simulink model "DualMIPS_sim2_amartya"  (R2025a)
settings: Solver=FixedStepDiscrete  StartTime=0  StopTime=200  FixedStep=1  RelTol=1e-3
libraries: simulink_extras x2, hdlsllib x2
settings Model: Creator=amartyaraoponugoti  LastModifiedBy=prath

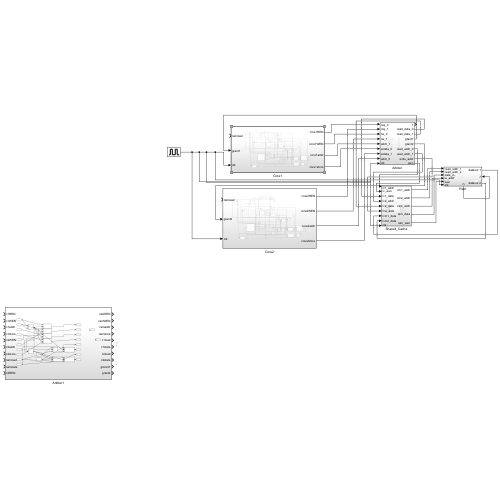
[thumbnail: Simulink's stored preview of the top-level diagram]
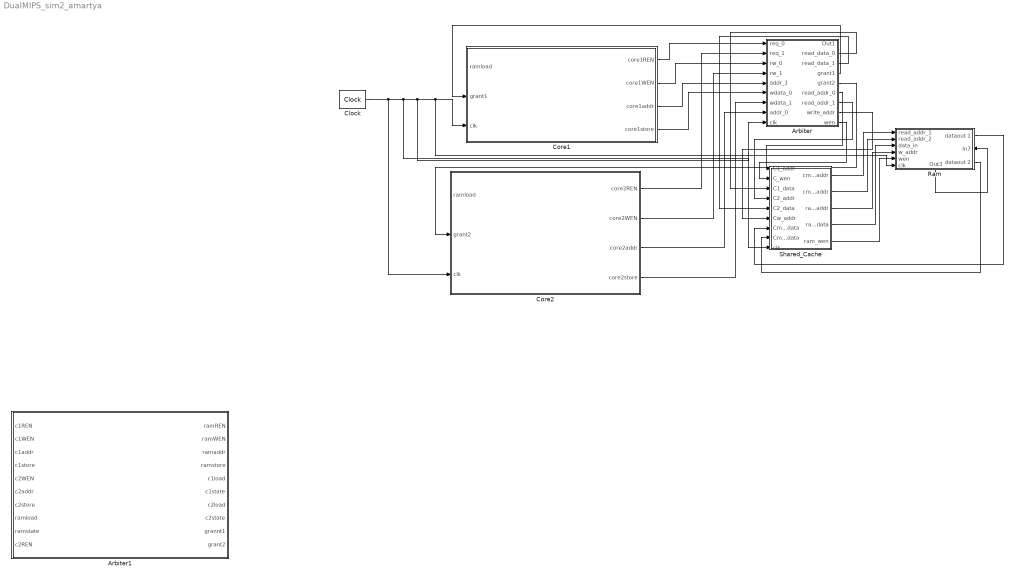
== system DualMIPS_sim2_amartya ==
  Arbiter : Subsystem
  Arbiter1 : Subsystem
  Clock : simulink_extras/Flip Flops/Clock  period=2
  Core1 : Subsystem
  Core2 : Subsystem
  Ram : Subsystem
      settings: PortSchema="{\"entries\":[{\"content\":{\"sides\":[{\"content\":{\"connectorIds\":[\"In1\",\"In2\",\"In3\",\"In4\",\"In5\",\"In6\"]},\"type\":\"ConnectorPlacement.EquallySpacedRectSide\",\"uuid\":\"e4753198-88eb-4d8c-8163-319740d05159\"},{\"content\":{\"connectorIds\":[\"Out1\",\"In7\",\"Out2\"],\"side\":\"RIGHT\"},\"type\":\"ConnectorPlacement.EquallySpacedRectSide\",\"uuid\":\"9705e5dc-da62-4ef6-ad04-f47eaed09c48\"},{\"content\":{\"side\":\"TOP\"},\"type\":\"ConnectorPlacement.EquallySpacedRectSide\",\"uuid\":\"34b411fe-a508-42ee-98a0-b8408ee3d948\"},{\"content\":{\"connectorIds\":[\"Out3\"],\"side\":\"BOTTOM\"},\"type\":\"ConnectorPlacement.EquallySpacedRectSide\",\"uuid\":\"02597b9b-60a8-49d4-9b54-171341e14a18\"}]},\"type\":\"ConnectorPlacement.EquallySpacedConnector\",\"uuid\":\"94fe3e38-0fe8-4e5d-a47f-3f60283f60e4\"}],\"packageUris\":[\"http://schema.mathworks.com/mf0/Connector/R2020b\"],\"version\":\"1.0\"}"
  Shared_Cache : Subsystem
  wires:
  Arbiter/4(grant1) -> Core1/2(grant1)
  Arbiter/5(grant2) -> Core2/2(grant2)
  Core1/1(core1REN) -> Arbiter/1(req_0)
  Core1/2(core1WEN) -> Arbiter/3(rw_0)
  Core1/3(core1addr) -> Arbiter/5(addr_1)
  Core1/4(core1store) -> Arbiter/6(wdata_0)
  Core2/1(core2REN) -> Arbiter/2(req_1)
  Core2/2(core2WEN) -> Arbiter/4(rw_1)
  Core2/3(core2addr) -> Arbiter/8(addr_0)
  Core2/4(core2store) -> Arbiter/7(wdata_1)
  Arbiter/6(read_addr_0) -> Shared_Cache/1(C1_addr)
  Arbiter/7(read_addr_1) -> Shared_Cache/4(C2_addr)
  Arbiter/2(read_data_0) -> Shared_Cache/3(C1_data)
  Arbiter/3(read_data_1) -> Shared_Cache/5(C2_data)
  Shared_Cache/5(ram_wen) -> Ram/5(wen)
  Shared_Cache/3(ram_addr) -> Ram/4(w_addr)
  Shared_Cache/4(ram_data) -> Ram/3(data_in)
  Shared_Cache/1(cm1_addr) -> Ram/1(read_addr_1)
  Shared_Cache/2(cm2_addr) -> Ram/2(read_addr_2)
  Ram/1(dataout 1) -> Shared_Cache/7(Cm1_data)
  Ram/2(dataout 2) -> Shared_Cache/8(Cm2_data)
  Arbiter/9(wen) -> Shared_Cache/2(C_wen)
  Arbiter/8(write_addr) -> Shared_Cache/6(Cw_addr)
  Clock/1 -> Core2/3(clk), Shared_Cache/9(clk), Arbiter/9(clk), Ram/6(clk), Core1/3(clk)
  Ram/3(Out3) -> Ram/7(In7)

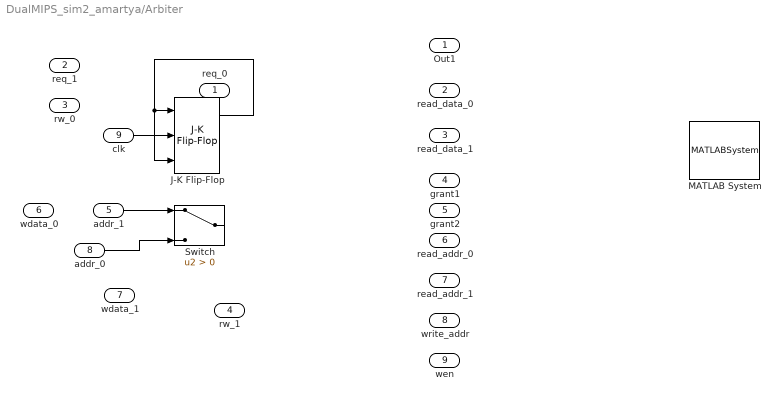
== system DualMIPS_sim2_amartya/Arbiter ==
  req_0 : Inport
  req_1 : Inport  Port=2
  rw_0 : Inport  Port=3
  rw_1 : Inport  Port=4
  addr_1 : Inport  Port=5
  wdata_0 : Inport  Port=6
  wdata_1 : Inport  Port=7
  addr_0 : Inport  Port=8
  clk : Inport  Port=9
  J-K Flip-Flop : simulink_extras/Flip Flops/J-K Flip-Flop  initial_condition=0
  MATLAB System : MATLABSystem
  Switch : Switch  Criteria=u2 > Threshold  SaturateOnIntegerOverflow=off  InputSameDT=off
  Out1 : Outport
  read_data_0 : Outport  Port=2
  read_data_1 : Outport  Port=3
  grant1 : Outport  Port=4
  grant2 : Outport  Port=5
  read_addr_0 : Outport  Port=6
  read_addr_1 : Outport  Port=7
  write_addr : Outport  Port=8
  wen : Outport  Port=9
  wires:
  clk/1 -> J-K Flip-Flop/2
  addr_1/1 -> Switch/1
  J-K Flip-Flop/1 -> J-K Flip-Flop/1, J-K Flip-Flop/3
  addr_0/1 -> Switch/3

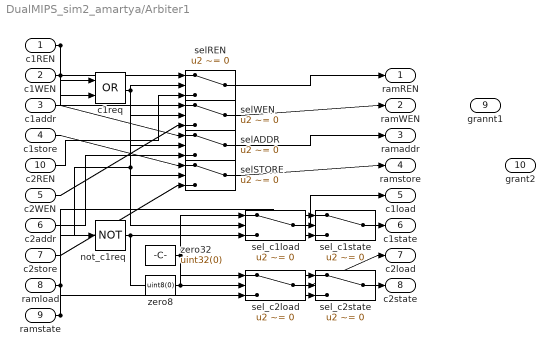
== system DualMIPS_sim2_amartya/Arbiter1 ==
  c1REN : Inport
  c1WEN : Inport  Port=2
  c1addr : Inport  Port=3
  c1store : Inport  Port=4
  c2WEN : Inport  Port=5
  c2addr : Inport  Port=6
  c2store : Inport  Port=7
  ramload : Inport  Port=8
  ramstate : Inport  Port=9
  c2REN : Inport  Port=10
  c1req : Logic  Operator=OR  AllPortsSameDT=off  OutDataTypeStr=boolean
  not_c1req : Logic  Operator=NOT  AllPortsSameDT=off  OutDataTypeStr=boolean
  selADDR : Switch  Criteria=u2 ~= 0  Threshold=0.5  SaturateOnIntegerOverflow=off  InputSameDT=off
  selREN : Switch  Criteria=u2 ~= 0  Threshold=0.5  SaturateOnIntegerOverflow=off  InputSameDT=off
  selSTORE : Switch  Criteria=u2 ~= 0  Threshold=0.5  SaturateOnIntegerOverflow=off  InputSameDT=off
  selWEN : Switch  Criteria=u2 ~= 0  Threshold=0.5  SaturateOnIntegerOverflow=off  InputSameDT=off
  sel_c1load : Switch  Criteria=u2 ~= 0  Threshold=0.5  SaturateOnIntegerOverflow=off  InputSameDT=off
  sel_c1state : Switch  Criteria=u2 ~= 0  Threshold=0.5  SaturateOnIntegerOverflow=off  InputSameDT=off
  sel_c2load : Switch  Criteria=u2 ~= 0  Threshold=0.5  SaturateOnIntegerOverflow=off  InputSameDT=off
  sel_c2state : Switch  Criteria=u2 ~= 0  Threshold=0.5  SaturateOnIntegerOverflow=off  InputSameDT=off
  zero32 : Constant  Value=uint32(0)
  zero8 : Constant  Value=uint8(0)
  ramREN : Outport
  ramWEN : Outport  Port=2
  ramaddr : Outport  Port=3
  ramstore : Outport  Port=4
  c1load : Outport  Port=5
  c1state : Outport  Port=6
  c2load : Outport  Port=7
  c2state : Outport  Port=8
  grannt1 : Outport  Port=9
  grant2 : Outport  Port=10
  wires:
  c1REN/1 -> c1req/1, selREN/1
  c1WEN/1 -> c1req/2, selWEN/1
  c1req/1 -> not_c1req/1, sel_c1load/2, sel_c1state/2, selREN/2, selWEN/2, selADDR/2, selSTORE/2
  c2REN/1 -> selREN/3
  c2WEN/1 -> selWEN/3
  c1addr/1 -> selADDR/1
  c2addr/1 -> selADDR/3
  c1store/1 -> selSTORE/1
  c2store/1 -> selSTORE/3
  selREN/1 -> ramREN/1
  selWEN/1 -> ramWEN/1
  selADDR/1 -> ramaddr/1
  selSTORE/1 -> ramstore/1
  zero32/1 -> sel_c1load/1, sel_c2load/1
  ramload/1 -> sel_c1load/3, sel_c2load/3
  sel_c1load/1 -> c1load/1
  not_c1req/1 -> sel_c2load/2, sel_c2state/2
  sel_c2load/1 -> c2load/1
  zero8/1 -> sel_c1state/1, sel_c2state/1
  ramstate/1 -> sel_c1state/3, sel_c2state/3
  sel_c1state/1 -> c1state/1
  sel_c2state/1 -> c2state/1

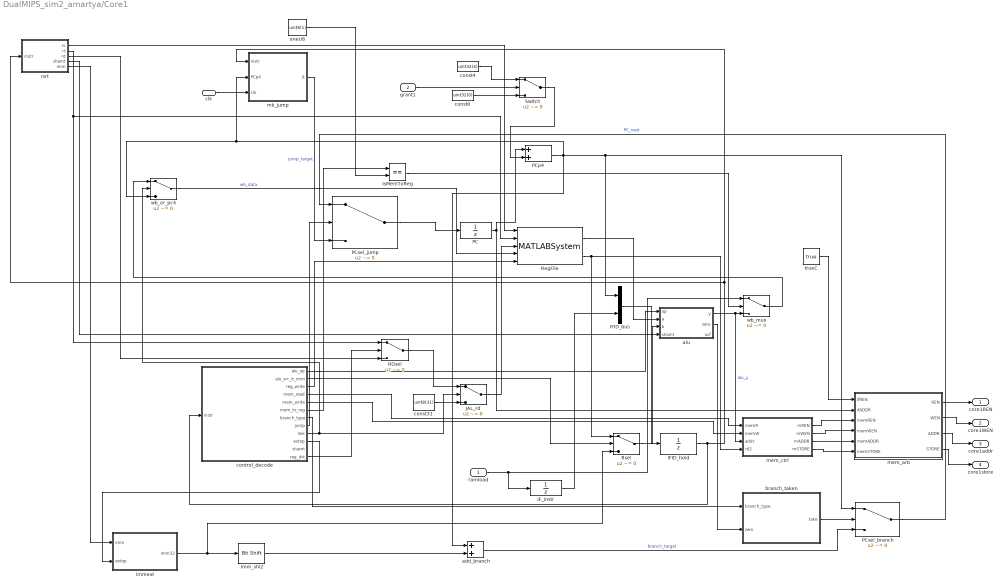
== system DualMIPS_sim2_amartya/Core1 ==
  ramload : Inport
  grant1 : Inport  Port=2
  clk : Inport  Port=3
  Bsel : Switch  Criteria=u2 ~= 0  SaturateOnIntegerOverflow=off  InputSameDT=off
  IFID_bus : BusCreator  Inputs=2
  IFID_hold : UnitDelay  SampleTime=-1  HasFrameUpgradeWarning=on
  IF_instr : UnitDelay  SampleTime=-1  HasFrameUpgradeWarning=on
  IsMemToReg : RelationalOperator  Operator===  OutDataTypeStr=boolean  RndMeth=Simplest  InputSameDT=off
  JAL_rd : Switch  Criteria=u2 ~= 0  SaturateOnIntegerOverflow=off  InputSameDT=off
  PC : UnitDelay  SampleTime=-1  HasFrameUpgradeWarning=on
  PCp4 : Sum
  PCsel_branch : Switch  Criteria=u2 ~= 0  SaturateOnIntegerOverflow=off  InputSameDT=off
  PCsel_jump : Switch  Criteria=u2 ~= 0  SaturateOnIntegerOverflow=off  InputSameDT=off
  RDsel : Switch  Criteria=u2 ~= 0  SaturateOnIntegerOverflow=off  InputSameDT=off
  RegFile : MATLABSystem  System=RegFileSys  SimulateUsing=Code generation
      mask Type: RegFileSys
  Switch : Switch  Criteria=u2 ~= 0  SaturateOnIntegerOverflow=off  InputSameDT=off
  add_branch : Sum
  alu : MATLAB Function  TreatAsAtomicUnit=on
  branch_taken : MATLAB Function  TreatAsAtomicUnit=on
  const0 : Constant  Value=uint32(0)
  const31 : Constant  Value=uint8(31)
  const4 : Constant  Value=uint32(4)
  control_decode : MATLAB Function  TreatAsAtomicUnit=on
  imm_shl2 : hdlsllib/Logic and Bit Operations/Bit Shift  mode=Shift Right Arithmetic  N=2
  immext : MATLAB Function  TreatAsAtomicUnit=on
  mem_arb : MATLAB Function  TreatAsAtomicUnit=on
  mem_ctrl : MATLAB Function  TreatAsAtomicUnit=on
  mk_jump : MATLAB Function  TreatAsAtomicUnit=on
  oneU8 : Constant  Value=uint8(1)
  rsrt : MATLAB Function  TreatAsAtomicUnit=on
  trueC : Constant  Value=true
  wb_mux : Switch  Criteria=u2 ~= 0  SaturateOnIntegerOverflow=off  InputSameDT=off
  wb_or_pc4 : Switch  Criteria=u2 ~= 0  SaturateOnIntegerOverflow=off  InputSameDT=off
  core1REN : Outport
  core1WEN : Outport  Port=2
  core1addr : Outport  Port=3
  core1store : Outport  Port=4
  wires:
  mem_arb/3(ADDR) -> core1addr/1
  mem_arb/2(WEN) -> core1WEN/1
  branch_taken/1(take) -> PCsel_branch/2
  mem_ctrl/3(mADDR) -> mem_arb/5(memADDR)
  mem_ctrl/1(mREN) -> mem_arb/3(memREN)
  RDsel/1 -> JAL_rd/1
  wb_mux/1 -> wb_or_pc4/1
  wb_or_pc4/1 -> RegFile/4  "wb_data"
  control_decode/9(link) -> JAL_rd/2, wb_or_pc4/2
  trueC/1 -> mem_arb/1(ifREN)
  Bsel/1 -> alu/3(b)
  IF_instr/1 -> IFID_bus/2
  IFID_hold/1 -> rsrt/1(instr), mk_jump/1(instr), control_decode/1(instr)
  add_branch/1 -> PCsel_branch/3  "branch_target"
  mem_ctrl/4(mSTORE) -> mem_arb/6(memSTORE)
  RegFile/1 -> alu/2(a)
  ramload/1 -> IF_instr/1, wb_mux/1
  JAL_rd/1 -> RegFile/3
  IFID_bus/1 -> IFID_hold/1
  const31/1 -> JAL_rd/3
  rsrt/4(shamt) -> alu/4(shamt)
  const4/1 -> Switch/1
  rsrt/1(rs) -> RegFile/1
  IsMemToReg/1 -> wb_mux/2
  mem_ctrl/2(mWEN) -> mem_arb/4(memWEN)
  imm_shl2/1 -> add_branch/2
  control_decode/10(extop) -> immext/2(extop)
  control_decode/6(mem_to_reg) -> IsMemToReg/1
  alu/2(zero) -> branch_taken/2(zero)
  control_decode/5(mem_write) -> mem_ctrl/2(memW)
  alu/1(y) -> mem_ctrl/3(addr), wb_mux/3  "alu_y"
  control_decode/4(mem_read) -> mem_ctrl/1(memR)
  mem_arb/1(REN) -> core1REN/1
  mem_arb/4(STORE) -> core1store/1
  control_decode/7(branch_type) -> branch_taken/1(branch_type)
  PCsel_branch/1 -> PCsel_jump/1  "PC_next"
  control_decode/3(reg_write) -> RegFile/5
  control_decode/1(alu_op) -> alu/1(op)
  PCp4/1 -> IFID_bus/1, PCsel_branch/1, wb_or_pc4/3, mk_jump/2(PCp4), add_branch/1
  mk_jump/1(jt) -> PCsel_jump/3  "jump_target"
  rsrt/2(rt) -> RegFile/2, RDsel/1
  immext/1(imm32) -> imm_shl2/1, Bsel/3
  control_decode/2(alu_src_b_imm) -> Bsel/2
  oneU8/1 -> IsMemToReg/2
  control_decode/12(reg_dst) -> RDsel/2
  rsrt/3(rd) -> RDsel/3
  PC/1 -> PCp4/1, mem_arb/2(ifADDR)
  control_decode/8(jump) -> PCsel_jump/2
  RegFile/2 -> Bsel/1, mem_ctrl/4(rd2)
  rsrt/5(imm) -> immext/1(imm)
  Switch/1 -> PCp4/2
  grant1/1 -> Switch/2
  const0/1 -> Switch/3
  clk/1 -> mk_jump/3(clk)
  PCsel_jump/1 -> PC/1

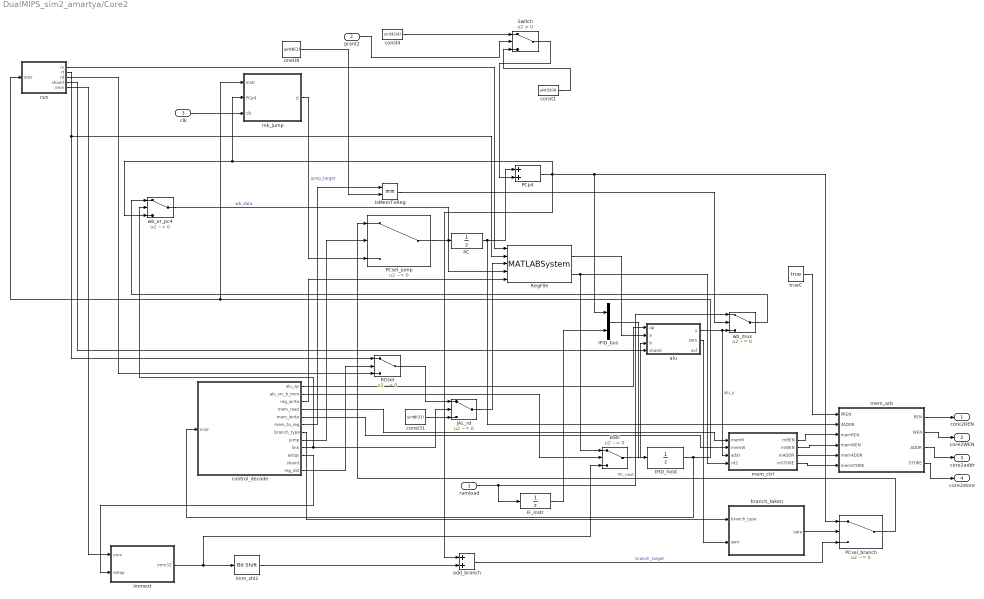
== system DualMIPS_sim2_amartya/Core2 ==
  ramload : Inport
  grant2 : Inport  Port=2
  clk : Inport  Port=3
  Bsel : Switch  Criteria=u2 ~= 0  SaturateOnIntegerOverflow=off  InputSameDT=off
  IFID_bus : BusCreator  Inputs=2
  IFID_hold : UnitDelay  SampleTime=-1  HasFrameUpgradeWarning=on
  IF_instr : UnitDelay  SampleTime=-1  HasFrameUpgradeWarning=on
  IsMemToReg : RelationalOperator  Operator===  OutDataTypeStr=boolean  RndMeth=Simplest  InputSameDT=off
  JAL_rd : Switch  Criteria=u2 ~= 0  SaturateOnIntegerOverflow=off  InputSameDT=off
  PC : UnitDelay  SampleTime=-1  HasFrameUpgradeWarning=on
  PCp4 : Sum
  PCsel_branch : Switch  Criteria=u2 ~= 0  SaturateOnIntegerOverflow=off  InputSameDT=off
  PCsel_jump : Switch  Criteria=u2 ~= 0  SaturateOnIntegerOverflow=off  InputSameDT=off
  RDsel : Switch  Criteria=u2 ~= 0  SaturateOnIntegerOverflow=off  InputSameDT=off
  RegFile : MATLABSystem  System=RegFileSys  SimulateUsing=Code generation
      mask Type: RegFileSys
  Switch : Switch  Criteria=u2 > Threshold  SaturateOnIntegerOverflow=off  InputSameDT=off
  add_branch : Sum
  alu : MATLAB Function  TreatAsAtomicUnit=on
  branch_taken : MATLAB Function  TreatAsAtomicUnit=on
  const1 : Constant  Value=uint32(4)
  const31 : Constant  Value=uint8(31)
  const4 : Constant  Value=uint32(4)
  control_decode : MATLAB Function  TreatAsAtomicUnit=on
  imm_shl2 : hdlsllib/Logic and Bit Operations/Bit Shift  mode=Shift Right Arithmetic  N=2
  immext : MATLAB Function  TreatAsAtomicUnit=on
  mem_arb : MATLAB Function  TreatAsAtomicUnit=on
  mem_ctrl : MATLAB Function  TreatAsAtomicUnit=on
  mk_jump : MATLAB Function  TreatAsAtomicUnit=on
  oneU8 : Constant  Value=uint8(1)
  rsrt : MATLAB Function  TreatAsAtomicUnit=on
  trueC : Constant  Value=true
  wb_mux : Switch  Criteria=u2 ~= 0  SaturateOnIntegerOverflow=off  InputSameDT=off
  wb_or_pc4 : Switch  Criteria=u2 ~= 0  SaturateOnIntegerOverflow=off  InputSameDT=off
  core2REN : Outport
  core2WEN : Outport  Port=2
  core2addr : Outport  Port=3
  core2store : Outport  Port=4
  wires:
  Switch/1 -> PCp4/2
  mem_ctrl/4(mSTORE) -> mem_arb/6(memSTORE)
  mem_arb/4(STORE) -> core2store/1
  IF_instr/1 -> IFID_bus/2
  mem_ctrl/2(mWEN) -> mem_arb/4(memWEN)
  IFID_bus/1 -> IFID_hold/1
  control_decode/10(extop) -> immext/2(extop)
  mem_arb/2(WEN) -> core2WEN/1
  IsMemToReg/1 -> wb_mux/2
  Bsel/1 -> alu/3(b)
  control_decode/2(alu_src_b_imm) -> Bsel/2
  RegFile/2 -> Bsel/1, mem_ctrl/4(rd2)
  control_decode/7(branch_type) -> branch_taken/1(branch_type)
  PCsel_branch/1 -> PCsel_jump/1  "PC_next"
  mk_jump/1(jt) -> PCsel_jump/3  "jump_target"
  wb_mux/1 -> wb_or_pc4/1
  control_decode/6(mem_to_reg) -> IsMemToReg/1
  mem_ctrl/3(mADDR) -> mem_arb/5(memADDR)
  trueC/1 -> mem_arb/1(ifREN)
  control_decode/3(reg_write) -> RegFile/5
  add_branch/1 -> PCsel_branch/3  "branch_target"
  mem_arb/3(ADDR) -> core2addr/1
  PCp4/1 -> IFID_bus/1, PCsel_branch/1, wb_or_pc4/3, mk_jump/2(PCp4), add_branch/1
  rsrt/5(imm) -> immext/1(imm)
  IFID_hold/1 -> rsrt/1(instr), mk_jump/1(instr), control_decode/1(instr)
  ramload/1 -> IF_instr/1, wb_mux/1
  alu/2(zero) -> branch_taken/2(zero)
  control_decode/4(mem_read) -> mem_ctrl/1(memR)
  control_decode/1(alu_op) -> alu/1(op)
  JAL_rd/1 -> RegFile/3
  alu/1(y) -> mem_ctrl/3(addr), wb_mux/3  "alu_y"
  control_decode/12(reg_dst) -> RDsel/2
  RegFile/1 -> alu/2(a)
  rsrt/4(shamt) -> alu/4(shamt)
  mem_arb/1(REN) -> core2REN/1
  wb_or_pc4/1 -> RegFile/4  "wb_data"
  rsrt/1(rs) -> RegFile/1
  rsrt/3(rd) -> RDsel/3
  mem_ctrl/1(mREN) -> mem_arb/3(memREN)
  PC/1 -> PCp4/1, mem_arb/2(ifADDR)
  control_decode/9(link) -> JAL_rd/2, wb_or_pc4/2
  control_decode/8(jump) -> PCsel_jump/2
  control_decode/5(mem_write) -> mem_ctrl/2(memW)
  oneU8/1 -> IsMemToReg/2
  RDsel/1 -> JAL_rd/1
  imm_shl2/1 -> add_branch/2
  rsrt/2(rt) -> RegFile/2, RDsel/1
  immext/1(imm32) -> imm_shl2/1, Bsel/3
  const31/1 -> JAL_rd/3
  branch_taken/1(take) -> PCsel_branch/2
  const4/1 -> Switch/1
  grant2/1 -> Switch/2
  const1/1 -> Switch/3
  PCsel_jump/1 -> PC/1
  clk/1 -> mk_jump/3(clk)

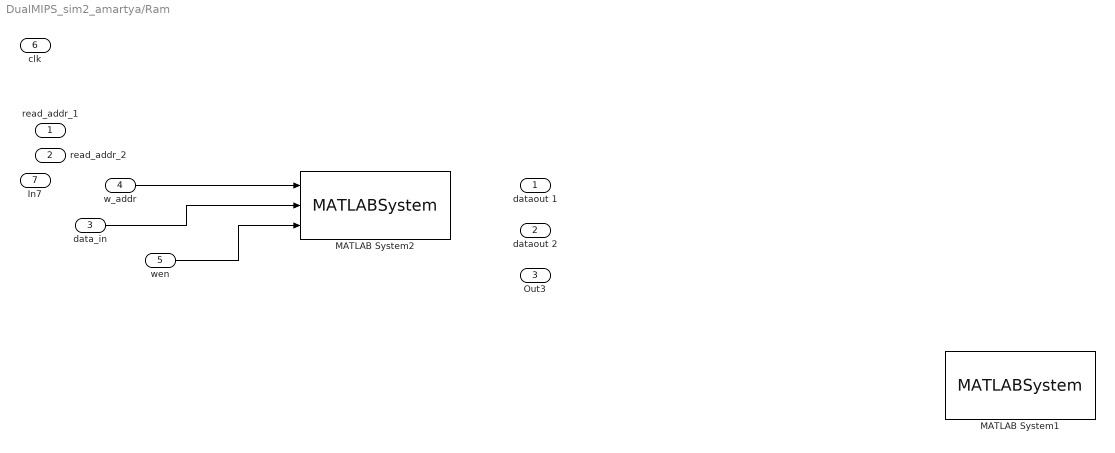
== system DualMIPS_sim2_amartya/Ram ==
  read_addr_1 : Inport
  read_addr_2 : Inport  Port=2
  data_in : Inport  Port=3
  w_addr : Inport  Port=4
  wen : Inport  Port=5
  clk : Inport  Port=6
  In7 : Inport  Port=7
  MATLAB System1 : MATLABSystem  System=RAMSys  Mem=zeros( 1024, 1, 'uint32' )  SimulateUsing=Code generation
      mask Type: RAMSys
  MATLAB System2 : MATLABSystem  System=RAMSys  Mem=zeros( 1024, 1, 'uint32' )  SimulateUsing=Code generation
      mask Type: RAMSys
  dataout 1 : Outport
  dataout 2 : Outport  Port=2
  Out3 : Outport  Port=3
  wires:
  wen/1 -> MATLAB System2/3
  data_in/1 -> MATLAB System2/2
  w_addr/1 -> MATLAB System2/1

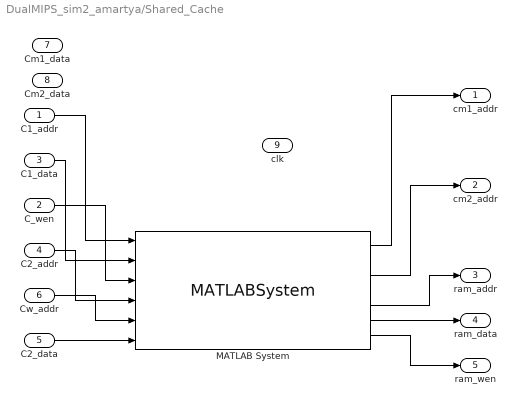
== system DualMIPS_sim2_amartya/Shared_Cache ==
  C1_addr : Inport
  C_wen : Inport  Port=2
  C1_data : Inport  Port=3
  C2_addr : Inport  Port=4
  C2_data : Inport  Port=5
  Cw_addr : Inport  Port=6
  Cm1_data : Inport  Port=7
  Cm2_data : Inport  Port=8
  clk : Inport  Port=9
  MATLAB System : MATLABSystem  System=SharedCacheSys  CacheData=zeros( 64, 1, 'uint32' )  CacheAddr=zeros( 64, 1, 'uint32' )  Valid=false( 64, 1 )  Dirty=false( 64, 1 )  SimulateUsing=Code generation
      mask Type: SharedCacheSys
  cm1_addr : Outport
  cm2_addr : Outport  Port=2
  ram_addr : Outport  Port=3
  ram_data : Outport  Port=4
  ram_wen : Outport  Port=5
  wires:
  Cw_addr/1 -> MATLAB System/5
  C1_addr/1 -> MATLAB System/1
  C1_data/1 -> MATLAB System/2
  MATLAB System/3 -> cm2_addr/1
  C_wen/1 -> MATLAB System/3
  C2_addr/1 -> MATLAB System/4
  MATLAB System/1 -> cm1_addr/1
  C2_data/1 -> MATLAB System/6
  MATLAB System/5 -> ram_addr/1
  MATLAB System/7 -> ram_wen/1
  MATLAB System/6 -> ram_data/1

== matlab function DualMIPS_sim2_amartya/Core1/mk_jump ==
  data: instr input; jt output; PCp4 input; clk input
function jt = mk_jump(instr, PCp4,clk)
% instr: current IFID_hold instruction
low26 = bitand(instr, uint32(hex2dec('03FFFFFF')));
low26sh2 = bitshift(low26, 2);
upper = bitand(PCp4, uint32(hex2dec('F0000000')));
jt = bitor(upper, low26sh2);
upper = bitand(clk, uint32(hex2dec('F0000000')));
jt = bitor(upper, low26sh2);
end

== matlab function DualMIPS_sim2_amartya/Core2/alu ==
  data: op input; y output; a input; b input; shamt input; zero output; ovf output
function [y, zero, ovf] = alu(op, a, b, shamt)
a = uint32(a); b = uint32(b); sa = int32(a); sb = int32(b);
switch uint8(op)
    case uint8(AluOp.ADD)
        tmp = uint64(a) + uint64(b);
        y = uint32(bitand(tmp, uint64(2^32-1)));
        ovf = tmp > uint64(2^32-1);
    case uint8(AluOp.SUB)
        tmp = int64(sa) - int64(sb);
        y = uint32(typecast(int32(tmp), 'uint32'));
        ovf = (tmp > int64(intmax('int32'))) || (tmp < int64(intmin('int32')));
    case uint8(AluOp.AND),  y = bitand(a,b); ovf=false;
    case uint8(AluOp.OR),   y = bitor(a,b);  ovf=false;
    case uint8(AluOp.XOR),  y = bitxor(a,b); ovf=false;
    case uint8(AluOp.NOR),  y = bitcmp(bitor(a,b),'uint32'); ovf=false;
    case uint8(AluOp.SLL),  y = bitshift(b, int16(shamt)); ovf=false;
    case uint8(AluOp.SRL),  y = bitshift(b, -int16(shamt)); ovf=false;
    case uint8(AluOp.SRA),  y = uint32(bitshift(sa, -int16(shamt))); ovf=false;
    case uint8(AluOp.SLT),  y = uint32(sa < sb); ovf=false;
    case uint8(AluOp.SLTU), y = uint32(a < b); ovf=false;
    case uint8(AluOp.PASSB),y = b; ovf=false;
    otherwise,              y = uint32(0); ovf=false;
end
zero = (y == 0);
end

== matlab function DualMIPS_sim2_amartya/Core2/branch_taken ==
  data: branch_type input; take output; zero input
function take = branch_taken(branch_type, zero)
% branch_type: 0=NONE, 1=BEQ, 2=BNE  (adjust if your enum differs)
take = false;
if branch_type == uint8(1)      % BEQ
    take = logical(zero);
elseif branch_type == uint8(2)  % BNE
    take = ~logical(zero);
end
end

== matlab function DualMIPS_sim2_amartya/Core2/control_decode ==
  data: instr input; alu_op output; alu_src_b_imm output; reg_write output; mem_read output; mem_write output; mem_to_reg output; branch_type output; jump output; link output; extop output; shamt output; reg_dst output
function [alu_op, alu_src_b_imm, reg_write, mem_read, mem_write, ...
          mem_to_reg, branch_type, jump, link, extop, shamt, reg_dst] = control_decode(instr)
% CONTROL_DECODE  One-instruction control for a MIPS-like core.
% Outputs:
%  mem_to_reg: 0=ALU, 1=Mem, 2=Link($ra)
%  jump: 0/1 (for J/JAL/JR)
%  branch_type: BranchType enum (NONE/BEQ/BNE/JR/J)
%
% instr must be uint32.

instr  = uint32(instr);

% --------- fields ----------
opcode = bitand(bitshift(instr,-26), uint32(63));     % [31:26]
funct  = bitand(instr,               uint32(63));     % [5:0]
shamt  = uint8(bitand(bitshift(instr,-6), uint32(31))); % [10:6]

% --------- defaults ----------
alu_op       = uint8(AluOp.ADD);
alu_src_b_imm= false;
reg_write    = false;
mem_read     = false;
mem_write    = false;
mem_to_reg   = uint8(0);     % 0:ALU, 1:Mem, 2:Link
branch_type  = uint8(BranchType.NONE);
jump         = uint8(0);
link         = false;
extop        = uint8(ExtOp.SIGNED);
reg_dst      = false;

is_Rtype = (opcode == 0);

if is_Rtype
    reg_dst   = true;
    switch uint32(funct)
        case 0,  alu_op=uint8(AluOp.SLL);  reg_write=true; % SLL
        case 2,  alu_op=uint8(AluOp.SRL);  reg_write=true; % SRL
        case 3,  alu_op=uint8(AluOp.SRA);  reg_write=true; % SRA
        case 32, alu_op=uint8(AluOp.ADD);  reg_write=true; % ADD
        case 33, alu_op=uint8(AluOp.ADD);  reg_write=true; % ADDU
        case 34, alu_op=uint8(AluOp.SUB);  reg_write=true; % SUB
        case 36, alu_op=uint8(AluOp.AND);  reg_write=true; % AND
        case 37, alu_op=uint8(AluOp.OR);   reg_write=true; % OR
        case 38, alu_op=uint8(AluOp.XOR);  reg_write=true; % XOR
        case 39, alu_op=uint8(AluOp.NOR);  reg_write=true; % NOR
        case 42, alu_op=uint8(AluOp.SLT);  reg_write=true; % SLT
        case 8   % JR
            branch_type = uint8(BranchType.JR);
            jump        = uint8(1);
            reg_write   = false;
        otherwise
            % NOP/unknown R-type
    end

else  % I/J type by opcode
    switch uint32(opcode)
        case 35  % LW
            alu_op=uint8(AluOp.ADD);  alu_src_b_imm=true;
            reg_write=true; mem_read=true; mem_to_reg=uint8(1);
        case 43  % SW
            alu_op=uint8(AluOp.ADD);  alu_src_b_imm=true; mem_write=true;
        case 4   % BEQ
            alu_op=uint8(AluOp.SUB);  branch_type=uint8(BranchType.BEQ);
        case 5   % BNE
            alu_op=uint8(AluOp.SUB);  branch_type=uint8(BranchType.BNE);
        case 8   % ADDI
            alu_op=uint8(AluOp.ADD);  alu_src_b_imm=true; reg_write=true;
        case 12  % ANDI
            alu_op=uint8(AluOp.AND);  alu_src_b_imm=true; reg_write=true; extop=uint8(ExtOp.UNSIGNED);
        case 13  % ORI
            alu_op=uint8(AluOp.OR);   alu_src_b_imm=true; reg_write=true; extop=uint8(ExtOp.UNSIGNED);
        case 15  % LUI
            alu_op=uint8(AluOp.PASSB); alu_src_b_imm=true; reg_write=true; extop=uint8(ExtOp.LUI);
        case 2   % J
            branch_type=uint8(BranchType.J); jump=uint8(1);
        case 3   % JAL
            branch_type=uint8(BranchType.J); jump=uint8(1);
            link=true; reg_write=true; mem_to_reg=uint8(2);
        otherwise
            % unknown/unsupported
    end
end
end

== matlab function DualMIPS_sim2_amartya/Core2/immext ==
  data: imm input; imm32 output; extop input
function imm32 = immext(imm,extop)
% extop: 0 SIGNED, 1 UNSIGNED, 2 LUI
if extop==2
    imm32 = bitshift(imm,16);
elseif extop==1
    imm32 = uint32(imm);
else
    % sign-extend 16 -> 32
    s = int32(typecast(uint16(imm),'int16'));
    imm32 = uint32(s);
end
end

== matlab function DualMIPS_sim2_amartya/Core2/mem_arb ==
  data: ifREN input; REN output; ifADDR input; memREN input; memWEN input; memADDR input; memSTORE input; WEN output; ADDR output; STORE output
function [REN,WEN,ADDR,STORE] = mem_arb(ifREN,ifADDR,memREN,memWEN,memADDR,memSTORE)
% IF side has priority over MEM side
if ifREN
    REN   = true;
    WEN   = false;
    ADDR  = ifADDR;
    STORE = uint32(0);
elseif memREN || memWEN
    REN   = memREN;
    WEN   = memWEN;
    ADDR  = memADDR;
    STORE = memSTORE;
else
    REN   = false;
    WEN   = false;
    ADDR  = uint32(0);
    STORE = uint32(0);
end
end

== matlab function DualMIPS_sim2_amartya/Core2/mem_ctrl ==
  data: memR input; mREN output; memW input; addr input; rd2 input; mWEN output; mADDR output; mSTORE output
function [mREN,mWEN,mADDR,mSTORE] = mem_ctrl(memR,memW,addr,rd2)
% memR: whether this instr is a load
% memW: whether this instr is a store
% addr: ALU result (address)
% rd2 : register file value to store

mREN   = memR;    % drives ramREN
mWEN   = memW;    % drives ramWEN
mADDR  = addr;    % drives ramaddr
mSTORE = rd2;     % drives ramstore
end

== matlab function DualMIPS_sim2_amartya/Core1/alu ==
  data: op input; y output; a input; b input; shamt input; zero output; ovf output
function [y, zero, ovf] = alu(op, a, b, shamt)
a = uint32(a); b = uint32(b); sa = int32(a); sb = int32(b);
switch uint8(op)
    case uint8(AluOp.ADD)
        tmp = uint64(a) + uint64(b);
        y = uint32(bitand(tmp, uint64(2^32-1)));
        ovf = tmp > uint64(2^32-1);
    case uint8(AluOp.SUB)
        tmp = int64(sa) - int64(sb);
        y = uint32(typecast(int32(tmp), 'uint32'));
        ovf = (tmp > int64(intmax('int32'))) || (tmp < int64(intmin('int32')));
    case uint8(AluOp.AND),  y = bitand(a,b); ovf=false;
    case uint8(AluOp.OR),   y = bitor(a,b);  ovf=false;
    case uint8(AluOp.XOR),  y = bitxor(a,b); ovf=false;
    case uint8(AluOp.NOR),  y = bitcmp(bitor(a,b),'uint32'); ovf=false;
    case uint8(AluOp.SLL),  y = bitshift(b, int16(shamt)); ovf=false;
    case uint8(AluOp.SRL),  y = bitshift(b, -int16(shamt)); ovf=false;
    case uint8(AluOp.SRA),  y = uint32(bitshift(sa, -int16(shamt))); ovf=false;
    case uint8(AluOp.SLT),  y = uint32(sa < sb); ovf=false;
    case uint8(AluOp.SLTU), y = uint32(a < b); ovf=false;
    case uint8(AluOp.PASSB),y = b; ovf=false;
    otherwise,              y = uint32(0); ovf=false;
end
zero = (y == 0);
end

== matlab function DualMIPS_sim2_amartya/Core2/mk_jump ==
  data: instr input; jt output; PCp4 input; clk input
function jt = mk_jump(instr, PCp4,clk)
% instr: current IFID_hold instruction
low26 = bitand(instr, uint32(hex2dec('03FFFFFF')));
low26sh2 = bitshift(low26, 2);
upper = bitand(PCp4, uint32(hex2dec('F0000000')));
jt = bitor(upper, low26sh2);
end

== matlab function DualMIPS_sim2_amartya/Core2/rsrt ==
  data: instr input; rs output; rt output; rd output; shamt output; imm output
function [rs,rt,rd,shamt,imm] = rsrt(instr)
rs = uint8(bitand(bitshift(instr,-21),uint32(31)));
rt = uint8(bitand(bitshift(instr,-16),uint32(31)));
rd = uint8(bitand(bitshift(instr,-11),uint32(31)));
shamt = uint8(bitand(bitshift(instr,-6),uint32(31)));
imm = uint32(bitand(instr,uint32(65535)));
end

== matlab function DualMIPS_sim2_amartya/Core1/control_decode ==
  data: instr input; alu_op output; alu_src_b_imm output; reg_write output; mem_read output; mem_write output; mem_to_reg output; branch_type output; jump output; link output; extop output; shamt output; reg_dst output
function [alu_op, alu_src_b_imm, reg_write, mem_read, mem_write, ...
          mem_to_reg, branch_type, jump, link, extop, shamt, reg_dst] = control_decode(instr)
% CONTROL_DECODE  One-instruction control for a MIPS-like core.
% Outputs:
%  mem_to_reg: 0=ALU, 1=Mem, 2=Link($ra)
%  jump: 0/1 (for J/JAL/JR)
%  branch_type: BranchType enum (NONE/BEQ/BNE/JR/J)
%
% instr must be uint32.

instr  = uint32(instr);

% --------- fields ----------
opcode = bitand(bitshift(instr,-26), uint32(63));     % [31:26]
funct  = bitand(instr,               uint32(63));     % [5:0]
shamt  = uint8(bitand(bitshift(instr,-6), uint32(31))); % [10:6]

% --------- defaults ----------
alu_op       = uint8(AluOp.ADD);
alu_src_b_imm= false;
reg_write    = false;
mem_read     = false;
mem_write    = false;
mem_to_reg   = uint8(0);     % 0:ALU, 1:Mem, 2:Link
branch_type  = uint8(BranchType.NONE);
jump         = uint8(0);
link         = false;
extop        = uint8(ExtOp.SIGNED);
reg_dst      = false;

is_Rtype = (opcode == 0);

if is_Rtype
    reg_dst   = true;
    switch uint32(funct)
        case 0,  alu_op=uint8(AluOp.SLL);  reg_write=true; % SLL
        case 2,  alu_op=uint8(AluOp.SRL);  reg_write=true; % SRL
        case 3,  alu_op=uint8(AluOp.SRA);  reg_write=true; % SRA
        case 32, alu_op=uint8(AluOp.ADD);  reg_write=true; % ADD
        case 33, alu_op=uint8(AluOp.ADD);  reg_write=true; % ADDU
        case 34, alu_op=uint8(AluOp.SUB);  reg_write=true; % SUB
        case 36, alu_op=uint8(AluOp.AND);  reg_write=true; % AND
        case 37, alu_op=uint8(AluOp.OR);   reg_write=true; % OR
        case 38, alu_op=uint8(AluOp.XOR);  reg_write=true; % XOR
        case 39, alu_op=uint8(AluOp.NOR);  reg_write=true; % NOR
        case 42, alu_op=uint8(AluOp.SLT);  reg_write=true; % SLT
        case 8   % JR
            branch_type = uint8(BranchType.JR);
            jump        = uint8(1);
            reg_write   = false;
        otherwise
            % NOP/unknown R-type
    end

else  % I/J type by opcode
    switch uint32(opcode)
        case 35  % LW
            alu_op=uint8(AluOp.ADD);  alu_src_b_imm=true;
            reg_write=true; mem_read=true; mem_to_reg=uint8(1);
        case 43  % SW
            alu_op=uint8(AluOp.ADD);  alu_src_b_imm=true; mem_write=true;
        case 4   % BEQ
            alu_op=uint8(AluOp.SUB);  branch_type=uint8(BranchType.BEQ);
        case 5   % BNE
            alu_op=uint8(AluOp.SUB);  branch_type=uint8(BranchType.BNE);
        case 8   % ADDI
            alu_op=uint8(AluOp.ADD);  alu_src_b_imm=true; reg_write=true;
        case 12  % ANDI
            alu_op=uint8(AluOp.AND);  alu_src_b_imm=true; reg_write=true; extop=uint8(ExtOp.UNSIGNED);
        case 13  % ORI
            alu_op=uint8(AluOp.OR);   alu_src_b_imm=true; reg_write=true; extop=uint8(ExtOp.UNSIGNED);
        case 15  % LUI
            alu_op=uint8(AluOp.PASSB); alu_src_b_imm=true; reg_write=true; extop=uint8(ExtOp.LUI);
        case 2   % J
            branch_type=uint8(BranchType.J); jump=uint8(1);
        case 3   % JAL
            branch_type=uint8(BranchType.J); jump=uint8(1);
            link=true; reg_write=true; mem_to_reg=uint8(2);
        otherwise
            % unknown/unsupported
    end
end
end

== matlab function DualMIPS_sim2_amartya/Core1/rsrt ==
  data: instr input; rs output; rt output; rd output; shamt output; imm output
function [rs,rt,rd,shamt,imm] = rsrt(instr)
rs = uint8(bitand(bitshift(instr,-21),uint32(31)));
rt = uint8(bitand(bitshift(instr,-16),uint32(31)));
rd = uint8(bitand(bitshift(instr,-11),uint32(31)));
shamt = uint8(bitand(bitshift(instr,-6),uint32(31)));
imm = uint32(bitand(instr,uint32(65535)));
end

== matlab function DualMIPS_sim2_amartya/Core1/immext ==
  data: imm input; imm32 output; extop input
function imm32 = immext(imm,extop)
% extop: 0 SIGNED, 1 UNSIGNED, 2 LUI
if extop==2
    imm32 = bitshift(imm,16);
elseif extop==1
    imm32 = uint32(imm);
else
    % sign-extend 16 -> 32
    s = int32(typecast(uint16(imm),'int16'));
    imm32 = uint32(s);
end
end

== matlab function DualMIPS_sim2_amartya/Core1/mem_ctrl ==
  data: memR input; mREN output; memW input; addr input; rd2 input; mWEN output; mADDR output; mSTORE output
function [mREN,mWEN,mADDR,mSTORE] = mem_ctrl(memR,memW,addr,rd2)
% memR: whether this instr is a load
% memW: whether this instr is a store
% addr: ALU result (address)
% rd2 : register file value to store

mREN   = memR;    % drives ramREN
mWEN   = memW;    % drives ramWEN
mADDR  = addr;    % drives ramaddr
mSTORE = rd2;     % drives ramstore
end

== matlab function DualMIPS_sim2_amartya/Core1/mem_arb ==
  data: ifREN input; REN output; ifADDR input; memREN input; memWEN input; memADDR input; memSTORE input; WEN output; ADDR output; STORE output
function [REN,WEN,ADDR,STORE] = mem_arb(ifREN,ifADDR,memREN,memWEN,memADDR,memSTORE)
% IF side has priority over MEM side
if ifREN
    REN   = true;
    WEN   = false;
    ADDR  = ifADDR;
    STORE = uint32(0);
elseif memREN || memWEN
    REN   = memREN;
    WEN   = memWEN;
    ADDR  = memADDR;
    STORE = memSTORE;
else
    REN   = false;
    WEN   = false;
    ADDR  = uint32(0);
    STORE = uint32(0);
end
end

== matlab function DualMIPS_sim2_amartya/Core1/branch_taken ==
  data: branch_type input; take output; zero input
function take = branch_taken(branch_type, zero)
% branch_type: 0=NONE, 1=BEQ, 2=BNE  (adjust if your enum differs)
take = false;
if branch_type == uint8(1)      % BEQ
    take = logical(zero);
elseif branch_type == uint8(2)  % BNE
    take = ~logical(zero);
end
end
